simulink model "closed_loop"  (R2019b)
settings: Solver=VariableStepAuto  StartTime=0.0  StopTime=10.0  RelTol=1e-3
values from neighbouring files (symbols this model uses):
  A = [[0 1 0]; [a_2/a_1 0 delta]; [-a_2/a_1 0 -M*gamma]]    [controller_tuning.m]
  Kd = 0.644    [controller_tuning.m]
  Ki = 61.92    [controller_tuning.m]
  Kp = 16.1    [controller_tuning.m]
  M = 0.0375    [controller_tuning.m]
undefined symbols (not defined in the file or in its folder): S
settings Model: Creator=leo  LastModifiedBy=leo

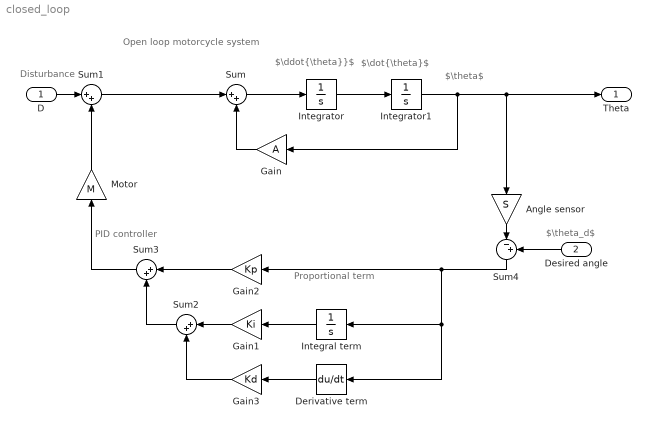
== system closed_loop ==
  note: $\theta_d$
  note: PID controller
  note: Proportional term
  note: Open loop motorcycle system
  note: Disturbance
  note: $\ddot{\theta}}$
  note: $\dot{\theta}$
  note: $\theta$
  "D " : Inport
  Desired angle : Inport  Port=2
  Angle sensor : Gain  Gain=S
  Derivative term : Derivative
  Gain : Gain  Gain=A
  Gain1 : Gain  Gain=Ki
  Gain2 : Gain  Gain=Kp
  Gain3 : Gain  Gain=Kd
  Integral term : Integrator
  Integrator : Integrator
  Integrator1 : Integrator
  Motor : Gain  Gain=M
  Sum{,1..3} (4 alike) : Sum  Inputs=|++
  Sum4 : Sum  Inputs=|-+
  Theta : Outport
  wires:
  "D "/1 -> Sum1/1
  Integrator1/1 -> Angle sensor/1, Theta/1, Gain/1
  Gain/1 -> Sum/2
  Sum/1 -> Integrator/1
  Integrator/1 -> Integrator1/1
  Sum1/1 -> Sum/1
  Gain2/1 -> Sum3/1
  Integral term/1 -> Gain1/1
  Derivative term/1 -> Gain3/1
  Sum4/1 -> Gain2/1, Derivative term/1, Integral term/1
  Gain1/1 -> Sum2/1
  Gain3/1 -> Sum2/2
  Sum2/1 -> Sum3/2
  Sum3/1 -> Motor/1
  Motor/1 -> Sum1/2
  Angle sensor/1 -> Sum4/1
  Desired angle/1 -> Sum4/2
